simulink model "volt_to_kelv"  (R2020b)
settings: Solver=VariableStepAuto  StartTime=0.0  StopTime=10.0  RelTol=1e-3
settings Model: Creator=Training  LastModifiedBy=Training

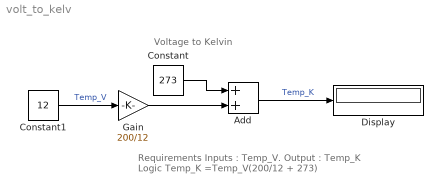
== system volt_to_kelv ==
  note: Requirements
      | Inputs : Temp_V.
      | Output : Temp_K
      | Logic
      | Temp_K =Temp_V(200/12 + 273)
  note: Voltage to Kelvin
  Add : Sum
  Constant : Constant  Value=273
  Constant1 : Constant  Value=12
  Display : Display
  Gain : Gain  Gain=200/12
  wires:
  Gain/1 -> Add/2
  Constant/1 -> Add/1
  Add/1 -> Display/1  "Temp_K"
  Constant1/1 -> Gain/1  "Temp_V"
